simulink model "BEV_PTC"  (R2023a)
settings: Solver=ode23tb  StartTime=0.0  StopTime=20e3  MaxStep=1  RelTol=1e-3
values from neighbouring files (symbols this model uses):
  mass = 20e3    (= 20000)    [run_BEV_simulations.m]    (also in run_FCHEV_simulations.m)
libraries: component_lib x67, slpidlib x6
settings Model: Creator=maxjo  LastModifiedBy=maxjo
settings SolverCC: ZeroCrossControl=DisableAll

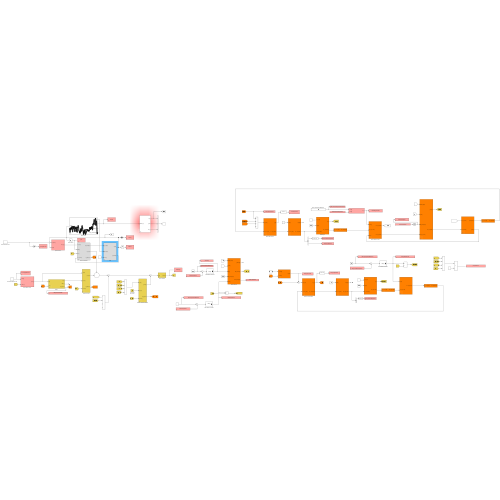
[thumbnail: Simulink's stored preview of the top-level diagram]
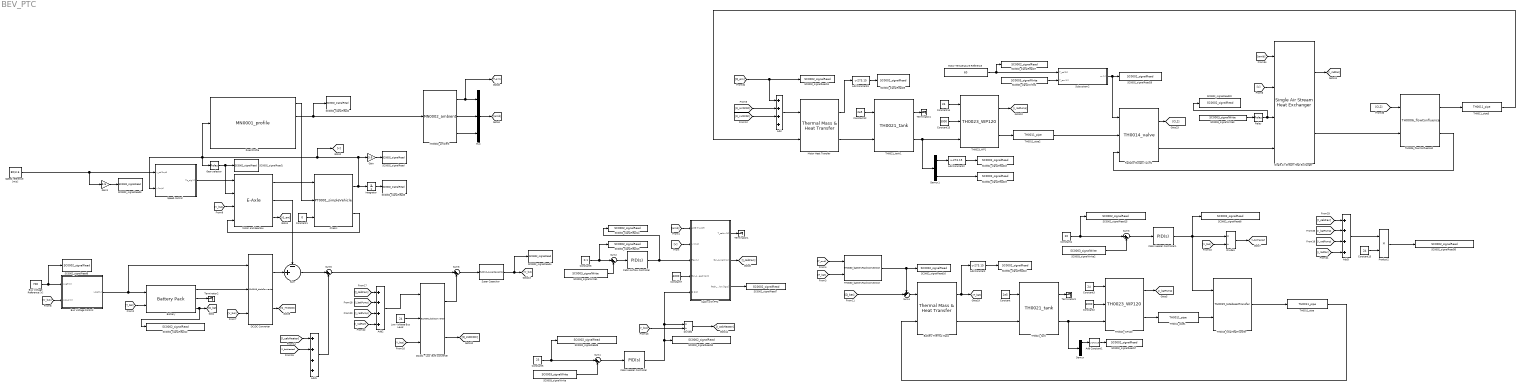
== system BEV_PTC ==
  Add{,1..3} (4 alike) : Sum  Inputs=++++
  Add Constant{,1..3} (4 alike) : Bias  Bias=-273.15  SaturateOnIntegerOverflow=off
  Battery : component_lib/Battery Pack  SOC_0=0.9  Nx=250  Ny=180
  Battery Thermal Mass : component_lib/Thermal Mass & Heat Transfer  n=100  d=10e-3  L=4  m=250 * 180 * 0.048  cp=1040  T_0=273 + 20
  Bus Voltage Control : Subsystem
  Bus Voltage Reference [V] : Constant  Value=700
  Cabin Airflow Controller : slpidlib/PID Controller  Controller=PID  Form=Parallel  TimeDomain=Continuous-time  UseExternalTs=off  SampleTime=-1  IntegratorMethod=Forward Euler  FilterMethod=Forward Euler  ControllerParametersSource=internal  P=1  I=1e-1  UseKiTs=off  D=0  N=100  UseFilter=on  TunerSelectOption=Transfer Function Based (PID Tuner App)  ZeroCross=off  InitialConditionSource=internal  InitialConditionForIntegrator=0.5  InitialConditionForFilter=0  DifferentiatorICPrevScaledInput=0  ExternalReset=none  TrackingMode=off  Kt=1  LimitOutput=on  SatLimitsSource=internal  UpperSaturationLimit=1  LowerSaturationLimit=0  LinearizeAsGain=on  AntiWindupMode=clamping  Kb=1  LimitIntegrator=off  UpperIntegratorSaturationLimit=inf  LowerIntegratorSaturationLimit=-inf  POutMin=[]  POutMax=[]  IOutMin=[]  IOutMax=[]  DOutMin=[]  DOutMax=[]  NOutMin=[]  NOutMax=[]  SumOutMin=[]  SumOutMax=[]  SaturationOutMin=[]  SaturationOutMax=[]  PParamMin=[]  PParamMax=[]  IParamMin=[]  IParamMax=[]  DParamMin=[]  DParamMax=[]  NParamMin=[]  NParamMax=[]  KbParamMin=[]  KbParamMax=[]  KtParamMin=[]  KtParamMax=[]  KbOutMin=[]  KbOutMax=[]  KtOutMin=[]  KtOutMax=[]  IntegratorOutMin=[]  IntegratorOutMax=[]  FilterOutMin=[]  FilterOutMax=[]  SumI1OutMin=[]  SumI1OutMax=[]  SumI2OutMin=[]  SumI2OutMax=[]  SumI3OutMin=[]  SumI3OutMax=[]  SumI4OutMin=[]  SumI4OutMax=[]  SumDOutMin=[]  SumDOutMax=[]  DifferentiatorOutMin=[]  DifferentiatorOutMax=[]  FilterDiffOutCoefMin=[]  FilterDiffOutCoefMax=[]  ReciprocalOutMin=[]  ReciprocalOutMax=[]  SumDenOutMin=[]  SumDenOutMax=[]  SumNumOutMin=[]  SumNumOutMax=[]  DivideOutMin=[]  DivideOutMax=[]  UdiffTsProdOutMin=[]  UdiffTsProdOutMax=[]  NTsProdOutMin=[]  NTsProdOutMax=[]  UintegralTsProdOutMin=[]  UintegralTsProdOutMax=[]  UngainTsProdOutMin=[]  UngainTsProdOutMax=[]  ClampingZeroOutDataTypeStr=Inherit: Inherit via back propagation  ClampingZeroOutMin=[]  ClampingZeroOutMax=[]  FilterDenConstantOutDataTypeStr=Inherit: Inherit via back propagation  FilterDenConstantOutMin=[]  FilterDenConstantOutMax=[]  PCopyOutDataTypeStr=Inherit: Inherit via back propagation  PCopyOutMin=[]  PCopyOutMax=[]  NCopyOutDataTypeStr=Inherit: Inherit via back propagation  NCopyOutMin=[]  NCopyOutMax=[]  IntegratorContinuousStateAttributes=''  IntegratorStateMustResolveToSignalObject=off  IntegratorRTWStateStorageClass=Auto  FilterContinuousStateAttributes=''  FilterStateMustResolveToSignalObject=off  FilterRTWStateStorageClass=Auto  ParallelPVariant=InternalParameters  IdealPVariant=Disabled  IVariant=InternalParameters  DVariant=InternalParameters  IntegratorVariant=Continuous  SatVariant=Enabled  AWVariant=ContClampingParallel  PCopyVariant=Disabled  TRVariant=Disabled  FdbkBlocksVariant=Forward  IdealPFdbkVariant=Disabled  SatFdbkVariant=Disabled  DerivativeFilterVariant=ContFilter  NVariant=InternalParameters  NCopyVariant=Disabled  FilterICVariant=InternalICsFilter  IntegratorICVariant=InternalICs  ExternalResetVariant=Disabled  TRSumVariant=Passthrough  SumFdbkVariant=Disabled  SumVariant=Sum_PID  TsampFilterVariant=InternalTs  TsampNgainVariant=Passthrough  TsampIntegralVariant=Disabled_SignalSpec  ExternalSaturationOutDataTypeStr=Inherit: Same as second input
  Cabin Heater Controller : slpidlib/PID Controller  Controller=PID  Form=Parallel  TimeDomain=Continuous-time  UseExternalTs=off  SampleTime=-1  IntegratorMethod=Forward Euler  FilterMethod=Forward Euler  ControllerParametersSource=internal  P=1e2  I=1e1  UseKiTs=off  D=0  N=100  UseFilter=on  TunerSelectOption=Transfer Function Based (PID Tuner App)  ZeroCross=off  InitialConditionSource=internal  InitialConditionForIntegrator=0  InitialConditionForFilter=0  DifferentiatorICPrevScaledInput=0  ExternalReset=none  TrackingMode=off  Kt=1  LimitOutput=on  SatLimitsSource=internal  UpperSaturationLimit=inf  LowerSaturationLimit=0  LinearizeAsGain=on  AntiWindupMode=clamping  Kb=1  LimitIntegrator=off  UpperIntegratorSaturationLimit=inf  LowerIntegratorSaturationLimit=-inf  POutMin=[]  POutMax=[]  IOutMin=[]  IOutMax=[]  DOutMin=[]  DOutMax=[]  NOutMin=[]  NOutMax=[]  SumOutMin=[]  SumOutMax=[]  SaturationOutMin=[]  SaturationOutMax=[]  PParamMin=[]  PParamMax=[]  IParamMin=[]  IParamMax=[]  DParamMin=[]  DParamMax=[]  NParamMin=[]  NParamMax=[]  KbParamMin=[]  KbParamMax=[]  KtParamMin=[]  KtParamMax=[]  KbOutMin=[]  KbOutMax=[]  KtOutMin=[]  KtOutMax=[]  IntegratorOutMin=[]  IntegratorOutMax=[]  FilterOutMin=[]  FilterOutMax=[]  SumI1OutMin=[]  SumI1OutMax=[]  SumI2OutMin=[]  SumI2OutMax=[]  SumI3OutMin=[]  SumI3OutMax=[]  SumI4OutMin=[]  SumI4OutMax=[]  SumDOutMin=[]  SumDOutMax=[]  DifferentiatorOutMin=[]  DifferentiatorOutMax=[]  FilterDiffOutCoefMin=[]  FilterDiffOutCoefMax=[]  ReciprocalOutMin=[]  ReciprocalOutMax=[]  SumDenOutMin=[]  SumDenOutMax=[]  SumNumOutMin=[]  SumNumOutMax=[]  DivideOutMin=[]  DivideOutMax=[]  UdiffTsProdOutMin=[]  UdiffTsProdOutMax=[]  NTsProdOutMin=[]  NTsProdOutMax=[]  UintegralTsProdOutMin=[]  UintegralTsProdOutMax=[]  UngainTsProdOutMin=[]  UngainTsProdOutMax=[]  ClampingZeroOutDataTypeStr=Inherit: Inherit via back propagation  ClampingZeroOutMin=[]  ClampingZeroOutMax=[]  FilterDenConstantOutDataTypeStr=Inherit: Inherit via back propagation  FilterDenConstantOutMin=[]  FilterDenConstantOutMax=[]  PCopyOutDataTypeStr=Inherit: Inherit via back propagation  PCopyOutMin=[]  PCopyOutMax=[]  NCopyOutDataTypeStr=Inherit: Inherit via back propagation  NCopyOutMin=[]  NCopyOutMax=[]  IntegratorContinuousStateAttributes=''  IntegratorStateMustResolveToSignalObject=off  IntegratorRTWStateStorageClass=Auto  FilterContinuousStateAttributes=''  FilterStateMustResolveToSignalObject=off  FilterRTWStateStorageClass=Auto  ParallelPVariant=InternalParameters  IdealPVariant=Disabled  IVariant=InternalParameters  DVariant=InternalParameters  IntegratorVariant=Continuous  SatVariant=Enabled  AWVariant=ContClampingParallel  PCopyVariant=Disabled  TRVariant=Disabled  FdbkBlocksVariant=Forward  IdealPFdbkVariant=Disabled  SatFdbkVariant=Disabled  DerivativeFilterVariant=ContFilter  NVariant=InternalParameters  NCopyVariant=Disabled  FilterICVariant=InternalICsFilter  IntegratorICVariant=InternalICs  ExternalResetVariant=Disabled  TRSumVariant=Passthrough  SumFdbkVariant=Disabled  SumVariant=Sum_PID  TsampFilterVariant=InternalTs  TsampNgainVariant=Passthrough  TsampIntegralVariant=Disabled_SignalSpec  ExternalSaturationOutDataTypeStr=Inherit: Same as second input
  Cabin Heater Controller1 : slpidlib/PID Controller  Controller=PID  Form=Parallel  TimeDomain=Continuous-time  UseExternalTs=off  SampleTime=-1  IntegratorMethod=Forward Euler  FilterMethod=Forward Euler  ControllerParametersSource=internal  P=1e2  I=1e1  UseKiTs=off  D=0  N=100  UseFilter=on  TunerSelectOption=Transfer Function Based (PID Tuner App)  ZeroCross=off  InitialConditionSource=internal  InitialConditionForIntegrator=0  InitialConditionForFilter=0  DifferentiatorICPrevScaledInput=0  ExternalReset=none  TrackingMode=off  Kt=1  LimitOutput=on  SatLimitsSource=internal  UpperSaturationLimit=inf  LowerSaturationLimit=0  LinearizeAsGain=on  AntiWindupMode=clamping  Kb=1  LimitIntegrator=off  UpperIntegratorSaturationLimit=inf  LowerIntegratorSaturationLimit=-inf  POutMin=[]  POutMax=[]  IOutMin=[]  IOutMax=[]  DOutMin=[]  DOutMax=[]  NOutMin=[]  NOutMax=[]  SumOutMin=[]  SumOutMax=[]  SaturationOutMin=[]  SaturationOutMax=[]  PParamMin=[]  PParamMax=[]  IParamMin=[]  IParamMax=[]  DParamMin=[]  DParamMax=[]  NParamMin=[]  NParamMax=[]  KbParamMin=[]  KbParamMax=[]  KtParamMin=[]  KtParamMax=[]  KbOutMin=[]  KbOutMax=[]  KtOutMin=[]  KtOutMax=[]  IntegratorOutMin=[]  IntegratorOutMax=[]  FilterOutMin=[]  FilterOutMax=[]  SumI1OutMin=[]  SumI1OutMax=[]  SumI2OutMin=[]  SumI2OutMax=[]  SumI3OutMin=[]  SumI3OutMax=[]  SumI4OutMin=[]  SumI4OutMax=[]  SumDOutMin=[]  SumDOutMax=[]  DifferentiatorOutMin=[]  DifferentiatorOutMax=[]  FilterDiffOutCoefMin=[]  FilterDiffOutCoefMax=[]  ReciprocalOutMin=[]  ReciprocalOutMax=[]  SumDenOutMin=[]  SumDenOutMax=[]  SumNumOutMin=[]  SumNumOutMax=[]  DivideOutMin=[]  DivideOutMax=[]  UdiffTsProdOutMin=[]  UdiffTsProdOutMax=[]  NTsProdOutMin=[]  NTsProdOutMax=[]  UintegralTsProdOutMin=[]  UintegralTsProdOutMax=[]  UngainTsProdOutMin=[]  UngainTsProdOutMax=[]  ClampingZeroOutDataTypeStr=Inherit: Inherit via back propagation  ClampingZeroOutMin=[]  ClampingZeroOutMax=[]  FilterDenConstantOutDataTypeStr=Inherit: Inherit via back propagation  FilterDenConstantOutMin=[]  FilterDenConstantOutMax=[]  PCopyOutDataTypeStr=Inherit: Inherit via back propagation  PCopyOutMin=[]  PCopyOutMax=[]  NCopyOutDataTypeStr=Inherit: Inherit via back propagation  NCopyOutMin=[]  NCopyOutMax=[]  IntegratorContinuousStateAttributes=''  IntegratorStateMustResolveToSignalObject=off  IntegratorRTWStateStorageClass=Auto  FilterContinuousStateAttributes=''  FilterStateMustResolveToSignalObject=off  FilterRTWStateStorageClass=Auto  ParallelPVariant=InternalParameters  IdealPVariant=Disabled  IVariant=InternalParameters  DVariant=InternalParameters  IntegratorVariant=Continuous  SatVariant=Enabled  AWVariant=ContClampingParallel  PCopyVariant=Disabled  TRVariant=Disabled  FdbkBlocksVariant=Forward  IdealPFdbkVariant=Disabled  SatFdbkVariant=Disabled  DerivativeFilterVariant=ContFilter  NVariant=InternalParameters  NCopyVariant=Disabled  FilterICVariant=InternalICsFilter  IntegratorICVariant=InternalICs  ExternalResetVariant=Disabled  TRSumVariant=Passthrough  SumFdbkVariant=Disabled  SumVariant=Sum_PID  TsampFilterVariant=InternalTs  TsampNgainVariant=Passthrough  TsampIntegralVariant=Disabled_SignalSpec  ExternalSaturationOutDataTypeStr=Inherit: Same as second input
  Cabin with PTC : Subsystem
  Chassi : component_lib/Powertrain/PT0001_simpleVehicle  m=mass  r_w=0.5  A_f=10  C_d=0.5  rho_air=1.225  c_r0=0.0060  c_r1=2.3e-7  gain=600  v0=75/3.6  x0=0
  Constant : Constant  Value=2e5
  Constant1 : Constant  Value=0
  Constant12 : Constant  Value=2e5
  Constant13 : Constant  Value=3000
  Constant14 : Constant  Value=24
  Constant15 : Constant  Value=24
  Constant2 : Constant  Value=3000
  Constant3 : Constant  Value=24
  Constant4 : Constant  Value=20
  Constant5 : Constant  Value=23
  Constant6 : Constant  Value=0.1
  Constant7 : Constant  Value=4000
  DC/DC - Low level converter : component_lib/Electrochemistry/EL0008_dcdcConverter  eta_up=0.98  eta_down=0.98
  DC/DC Converter : component_lib/Electrochemistry/EL0008_dcdcConverter  eta_up=0.99  eta_down=0.99
  Demux : Demux  Outputs=3
  Demux1 : Demux  Outputs=3
  Divide1 : Product  Inputs=*/
  Divide2 : Product  Inputs=*/
  Gain : Gain  Gain=3.6
  Gain1 : Gain  Gain=3.6
  Gear selector : Relay  OnSwitchValue=22  OffSwitchValue=21.5  OnOutputValue=4  OffOutputValue=3
  Integrator : Integrator
  Low Voltage Bus Level : Constant  Value=24
  MN0002_ambient : component_lib/Mission/MN0002_ambient  p_0=1.01e5  T_0=T_amb  RH_0=0.2
  Motor Heat Transfer : component_lib/Thermal Mass & Heat Transfer  n=100*4  d=10e-3  L=0.6  m=400  cp=420  T_0=273 + 70
  Motor Temperature Reference : Constant  Value=60
  Motor and Gearbox : component_lib/E-Axle  n=4  V_nom=700
  Mux : Mux  Inputs=3
  Product2 : Product
  Radiator Bypass Valve1 : component_lib/Thermal Systems/TH0014_valve  d=10e-2  dr=5e-2  C_d=0.9
  Relay : Relay  OnSwitchValue=85  OffSwitchValue=75  OnOutputValue=3000  ZeroCross=off
  Road Profile : component_lib/Mission/MN0001_profile  profile=Sodertalje_Norrkoping.mat  x0=0  N_lookahead=100
  SC0002_signalRead : component_lib/Data & Control/SC0002_signalRead  SigName=velocity
  SC0002_signalRead1 : component_lib/Data & Control/SC0002_signalRead  SigName=gear
  SC0002_signalRead10 : component_lib/Data & Control/SC0002_signalRead  SigName=cabinHeaterPower
  SC0002_signalRead11 : component_lib/Data & Control/SC0002_signalRead  SigName=motorGeneratedHeat
  SC0002_signalRead12 : component_lib/Data & Control/SC0002_signalRead  SigName=batteryGeneratedHeat
  SC0002_signalRead13 : component_lib/Data & Control/SC0002_signalRead  SigName=cabinFreshAirFlowReference
  SC0002_signalRead14 : component_lib/Data & Control/SC0002_signalRead  SigName=cabinFlap
  SC0002_signalRead15 : component_lib/Data & Control/SC0002_signalRead  SigName=batteryTemperatureReference
  SC0002_signalRead16 : component_lib/Data & Control/SC0002_signalRead  SigName=batteryConvection
  SC0002_signalRead17 : component_lib/Data & Control/SC0002_signalRead  SigName=batteryCoolantTemperature
  SC0002_signalRead18 : component_lib/Data & Control/SC0002_signalRead  SigName=radiatorCoolantTemperature
  SC0002_signalRead19 : component_lib/Data & Control/SC0002_signalRead  SigName=radiatorCoolantFlow
  SC0002_signalRead2 : component_lib/Data & Control/SC0002_signalRead  SigName=altitude
  SC0002_signalRead20 : component_lib/Data & Control/SC0002_signalRead  SigName=radiatorFanSpeed
  SC0002_signalRead22 : component_lib/Data & Control/SC0002_signalRead  SigName=batteryTemperature
  SC0002_signalRead25 : component_lib/Data & Control/SC0002_signalRead  SigName=motorTemperature
  SC0002_signalRead26 : component_lib/Data & Control/SC0002_signalRead  SigName=radiatorBypassValve
  SC0002_signalRead27 : component_lib/Data & Control/SC0002_signalRead  SigName=radiatorCoolantTemperatureReference
  SC0002_signalRead3 : component_lib/Data & Control/SC0002_signalRead  SigName=velocityReference
  SC0002_signalRead30 : component_lib/Data & Control/SC0002_signalRead  SigName=pumpfanPower
  SC0002_signalRead4 : component_lib/Data & Control/SC0002_signalRead  SigName=busVoltage
  SC0002_signalRead5 : component_lib/Data & Control/SC0002_signalRead  SigName=distance
  SC0002_signalRead6 : component_lib/Data & Control/SC0002_signalRead  SigName=busVoltageReference
  SC0002_signalRead7 : component_lib/Data & Control/SC0002_signalRead  SigName=cabinFreshAirFlow
  SC0002_signalRead8 : component_lib/Data & Control/SC0002_signalRead  SigName=batteryHeaterPower
  SC0002_signalRead9 : component_lib/Data & Control/SC0002_signalRead  SigName=cabinTemperatureReference
  SC0003_signalWrite : component_lib/Data & Control/SC0003_signalWrite  SigName=cabinTemperature
  SC0003_signalWrite1 : component_lib/Data & Control/SC0003_signalWrite  SigName=cabinFreshAirFlow
  SC0003_signalWrite2 : component_lib/Data & Control/SC0003_signalWrite  SigName=batteryCoolantTemperature
  SC0003_signalWrite3 : component_lib/Data & Control/SC0003_signalWrite  SigName=motorTemperature
  SC0003_signalWrite4 : component_lib/Data & Control/SC0003_signalWrite  SigName=radiatorCoolantTemperature
  Single Air Stream Heat Exchanger : component_lib/Single Air Stream Heat Exchanger  HtH=1.1  StS=0.95
  Speed control : Subsystem
  Speed reference [m/s] : Constant  Value=80/3.6
  Subsystem2 : Subsystem
  Sum : Sum  Inputs=-+|
  Sum{1..3,5..6} (5 alike) : Sum  Inputs=|+-
  Sum4 : Sum  Inputs=++|
  Super Capacitor : component_lib/Electrochemistry/EL0010_superCapacitor  C=100  V_bus0=700
  TH0006_flowConfluence2 : component_lib/Thermal Systems/TH0006_flowConfluence  gain=0.01
  TH0011_pipe : component_lib/Thermal Systems/TH0011_pipe  d=19e-3  L=5  e=0.006e-3  T_0=273 + 20
  TH0011_pipe1 : component_lib/Thermal Systems/TH0011_pipe  d=19e-3  L=2  e=0.006e-3  T_0=273 + 20
  TH0011_pipe2 : component_lib/Thermal Systems/TH0011_pipe  d=19e-3  L=2  e=0.006e-3  T_0=273 + 20
  TH0011_pipe3 : component_lib/Thermal Systems/TH0011_pipe  d=19e-3  L=5  e=0.006e-3  T_0=273 + 20
  TH0015_totalHeatTransfer : component_lib/Thermal Systems/TH0015_totalHeatTransfer  T_max=273+100  T_min=273
  TH0021_tank : component_lib/Thermal Systems/TH0021_tank  V=5e-3  T0=273.15 + 25
  TH0021_tank1 : component_lib/Thermal Systems/TH0021_tank  V=5e-3  T0=273.15 + 25
  TH0023_WP1 : component_lib/Thermal Systems/TH0023_WP120  SystemSampleTime=-1  VariantActivationTime=update diagram  Latency=0  AutoFrameSizeCalculation=off
  TH0023_WP120 : component_lib/Thermal Systems/TH0023_WP120  SystemSampleTime=-1  VariantActivationTime=update diagram  Latency=0  AutoFrameSizeCalculation=off
  TH0030_batteryPackConvection : component_lib/Thermal Systems/TH0030_batteryPackConvection  A=2*10  h=8
  Terminator{1..4} (4 alike) : Terminator
  wires:
  Speed reference [m/s]/1 -> Speed control/1(v_ref [m/s]), Gain1/1
  Motor and Gearbox/2 -> Sum/1
  Bus Voltage Reference [V]/1 -> Bus Voltage Control/1(V_ref [V]), SC0002_signalRead6/1
  Chassi/1 -> Integrator/1, Gain/1, [v], Speed control/2(v [m/s]), Road Profile/1, Gear selector/1
  Battery/2 -> Terminator2/1
  Motor and Gearbox/1 -> Chassi/1
  DC/DC Converter/1 -> Sum/2
  Road Profile/1 -> Chassi/2
  Road Profile/2 -> MN0002_ambient/1, SC0002_signalRead2/1
  Constant1/1 -> Chassi/3
  [T_bat] -> Battery/2
  Gain/1 -> SC0002_signalRead/1
  Gear selector/1 -> Motor and Gearbox/2, SC0002_signalRead1/1
  Gain1/1 -> SC0002_signalRead3/1
  Chassi/2 -> Motor and Gearbox/4
  Bus Voltage Control/1(I_bat [-]) -> DC/DC Converter/1, Battery/1
  Integrator/1 -> SC0002_signalRead5/1
  Speed control/1(Tq_sig [-]) -> Motor and Gearbox/1
  Super Capacitor/1 -> [V_bus], SC0002_signalRead4/1
  Battery/1 -> DC/DC Converter/2
  Battery/3 -> SC0002_signalRead12/1, [Q_bat]
  Motor and Gearbox/3 -> [Q_em]
  Cabin Airflow Controller/1 -> Cabin with PTC/3(flap [-]), SC0002_signalRead14/1
  Constant7/1 -> Cabin with PTC/4(fan_speed [rpm])
  [v] -> Cabin with PTC/2(v [m/s])
  MN0002_ambient/3 -> Mux/3
  MN0002_ambient/1 -> [T_amb], Mux/1
  MN0002_ambient/2 -> Mux/2
  Mux/1 -> [amb]
  [amb] -> Cabin with PTC/1(AMB (T,p,RH))
  Cabin with PTC/3(fresh_flow [kg/s]) -> SC0002_signalRead7/1
  Constant5/1 -> Sum1/1, SC0002_signalRead9/1
  SC0003_signalWrite/1 -> Sum1/2
  Sum1/1 -> Cabin Heater Controller/1
  SC0003_signalWrite1/1 -> Sum2/2
  Sum2/1 -> Cabin Airflow Controller/1
  Constant6/1 -> Sum2/1, SC0002_signalRead13/1
  Cabin with PTC/1(T_cabin [K]) -> Terminator1/1
  Cabin with PTC/2(fan_current [A]) -> [I_cabFan]
  Cabin Heater Controller/1 -> Divide2/1, Cabin with PTC/5(Q [J/s]), SC0002_signalRead10/1
  Battery Thermal Mass/1 -> [T_bat], Add Constant/1
  TH0015_totalHeatTransfer/1 -> TH0011_pipe/1
  TH0011_pipe1/1 -> TH0015_totalHeatTransfer/2
  Constant/1 -> TH0021_tank/1
  TH0021_tank/2 -> Demux/1, TH0023_WP120/3
  TH0023_WP120/2 -> TH0011_pipe1/1
  Battery Thermal Mass/2 -> TH0021_tank/2
  Constant2/1 -> TH0023_WP120/2
  Constant3/1 -> TH0023_WP120/1
  TH0023_WP120/1 -> [I_batPump]
  SC0003_signalWrite2/1 -> Sum3/2
  Divide1/1 -> [I_batHeater]
  Cabin Heater Controller1/1 -> SC0002_signalRead8/1, TH0015_totalHeatTransfer/1, Divide1/1
  Sum3/1 -> Cabin Heater Controller1/1
  Constant4/1 -> Sum3/1, SC0002_signalRead15/1
  TH0021_tank/1 -> Terminator3/1
  Add Constant/1 -> SC0002_signalRead22/1
  [T_bat] -> TH0030_batteryPackConvection/2
  [T_amb] -> TH0030_batteryPackConvection/1
  [Q_bat] -> Sum4/2
  Sum4/1 -> Battery Thermal Mass/1
  TH0030_batteryPackConvection/1 -> SC0002_signalRead16/1, Sum4/1
  TH0011_pipe/1 -> Battery Thermal Mass/2
  Demux/1 -> Add Constant1/1
  Add Constant1/1 -> SC0002_signalRead17/1
  Radiator Bypass Valve1/1 -> [CL2]
  [CL2] -> TH0006_flowConfluence2/1
  [amb] -> Single Air Stream Heat Exchanger/1
  Motor Temperature Reference/1 -> SC0002_signalRead27/1, Subsystem2/1(T_ref [K])
  TH0011_pipe3/1 -> Motor Heat Transfer/2
  Subsystem2/1(cv [-]) -> Radiator Bypass Valve1/1, SC0002_signalRead26/1
  SC0003_signalWrite4/1 -> Subsystem2/2(T_em [K])
  TH0011_pipe2/1 -> Radiator Bypass Valve1/2
  Motor Heat Transfer/1 -> Add Constant3/1
  DC/DC Converter/2 -> [Q_HVDCDC]
  TH0023_WP1/2 -> TH0011_pipe2/1
  Add Constant2/1 -> SC0002_signalRead18/1
  Constant12/1 -> TH0021_tank1/1
  Constant14/1 -> TH0023_WP1/1
  TH0021_tank1/1 -> Terminator4/1
  TH0021_tank1/2 -> Demux1/1, TH0023_WP1/3
  TH0023_WP1/1 -> [I_radPump]
  Constant13/1 -> TH0023_WP1/2
  Demux1/1 -> Add Constant2/1
  Motor Heat Transfer/2 -> TH0021_tank1/2
  Add Constant3/1 -> SC0002_signalRead25/1
  TH0006_flowConfluence2/2 -> Radiator Bypass Valve1/3
  Radiator Bypass Valve1/2 -> Single Air Stream Heat Exchanger/4
  Single Air Stream Heat Exchanger/2 -> TH0006_flowConfluence2/2
  [v] -> Single Air Stream Heat Exchanger/2
  Single Air Stream Heat Exchanger/1 -> [I_radFan]
  Demux1/3 -> SC0002_signalRead19/1
  Relay/1 -> SC0002_signalRead20/1, Single Air Stream Heat Exchanger/3
  SC0003_signalWrite3/1 -> Relay/1
  [Q_em] -> SC0002_signalRead11/1, Add/1
  [V_bus] -> DC/DC - Low level converter/3
  Low Voltage Bus Level/1 -> DC/DC - Low level converter/2
  DC/DC - Low level converter/1 -> Sum6/2
  DC/DC - Low level converter/2 -> [Q_LVDCDC]
  Sum6/1 -> Super Capacitor/1
  [V_bus] -> DC/DC Converter/3
  [V_bus] -> Bus Voltage Control/2(V_bus [V])
  [V_bus] -> Motor and Gearbox/3
  Add/1 -> Motor Heat Transfer/1
  [Q_HVDCDC] -> Add/2
  [Q_LVDCDC] -> Add/3
  [V_bus] -> Divide1/2
  [V_bus] -> Divide2/2
  Divide2/1 -> [I_cabHeater]
  Sum/1 -> Sum5/1
  Sum5/1 -> Sum6/1
  Add1/1 -> Sum5/2
  [I_cabHeater] -> Add1/1
  [I_batHeater] -> Add1/2
  Add2/1 -> DC/DC - Low level converter/1
  [I_cabFan] -> Add2/1
  [I_batPump] -> Add2/2
  Add3/1 -> Product2/1
  [I_radPump] -> Add3/3
  [I_cabFan] -> Add3/1
  Product2/1 -> SC0002_signalRead30/1
  Constant15/1 -> Product2/2
  [I_batPump] -> Add3/2
  [I_radPump] -> Add2/3
  TH0006_flowConfluence2/1 -> TH0011_pipe3/1
  [I_radFan] -> Add3/4
  [I_radFan] -> Add2/4

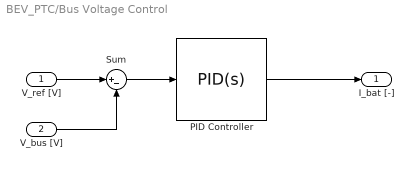
== system BEV_PTC/Bus Voltage Control ==
  V_ref [V] : Inport
  V_bus [V] : Inport  Port=2
  PID Controller : slpidlib/PID Controller  Controller=PID  Form=Parallel  TimeDomain=Continuous-time  UseExternalTs=off  SampleTime=-1  IntegratorMethod=Forward Euler  FilterMethod=Forward Euler  ControllerParametersSource=internal  P=1e2  I=1  UseKiTs=off  D=0  N=100  UseFilter=on  TunerSelectOption=Transfer Function Based (PID Tuner App)  ZeroCross=off  InitialConditionSource=internal  InitialConditionForIntegrator=0  InitialConditionForFilter=0  DifferentiatorICPrevScaledInput=0  ExternalReset=none  TrackingMode=off  Kt=1  LimitOutput=on  SatLimitsSource=internal  UpperSaturationLimit=725*2  LowerSaturationLimit=-725  LinearizeAsGain=on  AntiWindupMode=clamping  Kb=1  LimitIntegrator=off  UpperIntegratorSaturationLimit=inf  LowerIntegratorSaturationLimit=-inf  POutMin=[]  POutMax=[]  IOutMin=[]  IOutMax=[]  DOutMin=[]  DOutMax=[]  NOutMin=[]  NOutMax=[]  SumOutMin=[]  SumOutMax=[]  SaturationOutMin=[]  SaturationOutMax=[]  PParamMin=[]  PParamMax=[]  IParamMin=[]  IParamMax=[]  DParamMin=[]  DParamMax=[]  NParamMin=[]  NParamMax=[]  KbParamMin=[]  KbParamMax=[]  KtParamMin=[]  KtParamMax=[]  KbOutMin=[]  KbOutMax=[]  KtOutMin=[]  KtOutMax=[]  IntegratorOutMin=[]  IntegratorOutMax=[]  FilterOutMin=[]  FilterOutMax=[]  SumI1OutMin=[]  SumI1OutMax=[]  SumI2OutMin=[]  SumI2OutMax=[]  SumI3OutMin=[]  SumI3OutMax=[]  SumI4OutMin=[]  SumI4OutMax=[]  SumDOutMin=[]  SumDOutMax=[]  DifferentiatorOutMin=[]  DifferentiatorOutMax=[]  FilterDiffOutCoefMin=[]  FilterDiffOutCoefMax=[]  ReciprocalOutMin=[]  ReciprocalOutMax=[]  SumDenOutMin=[]  SumDenOutMax=[]  SumNumOutMin=[]  SumNumOutMax=[]  DivideOutMin=[]  DivideOutMax=[]  UdiffTsProdOutMin=[]  UdiffTsProdOutMax=[]  NTsProdOutMin=[]  NTsProdOutMax=[]  UintegralTsProdOutMin=[]  UintegralTsProdOutMax=[]  UngainTsProdOutMin=[]  UngainTsProdOutMax=[]  ClampingZeroOutDataTypeStr=Inherit: Inherit via back propagation  ClampingZeroOutMin=[]  ClampingZeroOutMax=[]  FilterDenConstantOutDataTypeStr=Inherit: Inherit via back propagation  FilterDenConstantOutMin=[]  FilterDenConstantOutMax=[]  PCopyOutDataTypeStr=Inherit: Inherit via back propagation  PCopyOutMin=[]  PCopyOutMax=[]  NCopyOutDataTypeStr=Inherit: Inherit via back propagation  NCopyOutMin=[]  NCopyOutMax=[]  IntegratorContinuousStateAttributes=''  IntegratorStateMustResolveToSignalObject=off  IntegratorRTWStateStorageClass=Auto  FilterContinuousStateAttributes=''  FilterStateMustResolveToSignalObject=off  FilterRTWStateStorageClass=Auto  ParallelPVariant=InternalParameters  IdealPVariant=Disabled  IVariant=InternalParameters  DVariant=InternalParameters  IntegratorVariant=Continuous  SatVariant=Enabled  AWVariant=ContClampingParallel  PCopyVariant=Disabled  TRVariant=Disabled  FdbkBlocksVariant=Forward  IdealPFdbkVariant=Disabled  SatFdbkVariant=Disabled  DerivativeFilterVariant=ContFilter  NVariant=InternalParameters  NCopyVariant=Disabled  FilterICVariant=InternalICsFilter  IntegratorICVariant=InternalICs  ExternalResetVariant=Disabled  TRSumVariant=Passthrough  SumFdbkVariant=Disabled  SumVariant=Sum_PID  TsampFilterVariant=InternalTs  TsampNgainVariant=Passthrough  TsampIntegralVariant=Disabled_SignalSpec  ExternalSaturationOutDataTypeStr=Inherit: Same as second input
  Sum : Sum  Inputs=|+-
  I_bat [-] : Outport
  wires:
  PID Controller/1 -> I_bat [-]/1
  Sum/1 -> PID Controller/1
  V_ref [V]/1 -> Sum/1
  V_bus [V]/1 -> Sum/2

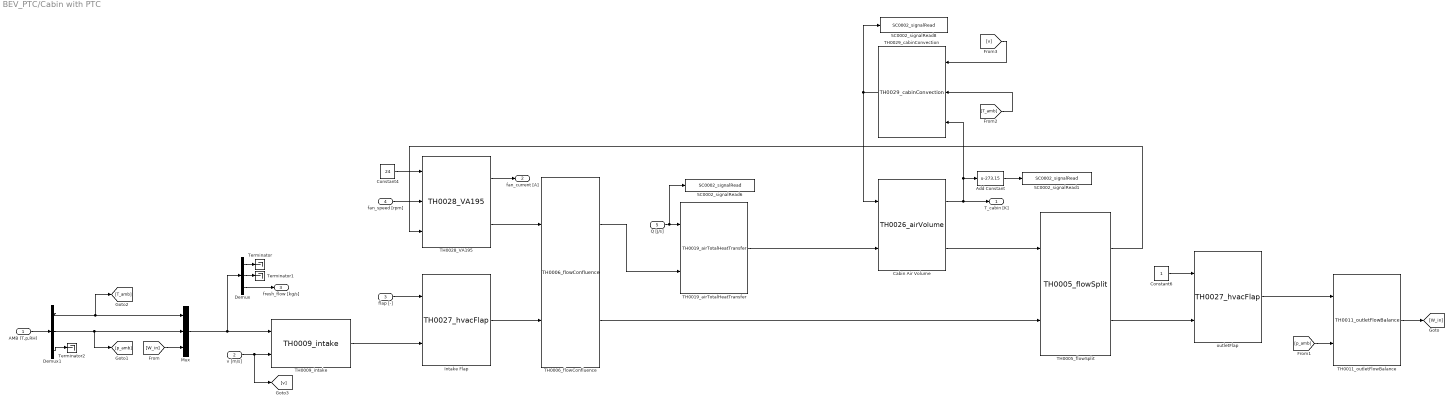
== system BEV_PTC/Cabin with PTC ==
  AMB (T,p,RH) : Inport
  v [m/s] : Inport  Port=2
  flap [-] : Inport  Port=3
  fan_speed [rpm] : Inport  Port=4
  Q [J/s] : Inport  Port=5
  Add Constant : Bias  Bias=-273.15  SaturateOnIntegerOverflow=off
  Cabin Air Volume : component_lib/Thermal Systems/TH0026_airVolume  V=4  T0=273.15 + 20
  Constant4 : Constant  Value=24
  Constant6 : Constant
  Demux : Demux  Outputs=3
  Demux1 : Demux  Outputs=3
  Intake Flap : component_lib/Thermal Systems/TH0027_hvacFlap  A=0.04  zeta=0.3
  Mux : Mux  Inputs=3
  SC0002_signalRead1 : component_lib/Data & Control/SC0002_signalRead  SigName=cabinTemperature
  SC0002_signalRead6 : component_lib/Data & Control/SC0002_signalRead  SigName=cabinHeating
  SC0002_signalRead8 : component_lib/Data & Control/SC0002_signalRead  SigName=cabinConvection
  TH0005_flowSplit : component_lib/Thermal Systems/TH0005_flowSplit  SystemSampleTime=-1  VariantActivationTime=update diagram  Latency=0  AutoFrameSizeCalculation=off
  TH0006_flowConfluence : component_lib/Thermal Systems/TH0006_flowConfluence  gain=0.01
  TH0009_intake : component_lib/Thermal Systems/TH0009_intake  zeta=0.1
  TH0011_outletFlowBalance : component_lib/Thermal Systems/TH0011_outletFlowBalance  gain=0.05
  TH0019_airTotalHeatTransfer : component_lib/Thermal Systems/TH0019_airTotalHeatTransfer  T_min=273-40  T_max=273+140
  TH0028_VA195 : component_lib/Thermal Systems/TH0028_VA195  n=1
      settings: LibrarySourceBlock=component_lib/Thermal Systems/TH0023_WP120
  TH0029_cabinConvection : component_lib/Thermal Systems/TH0029_cabinConvection  A=2
  Terminator : Terminator
  Terminator1 : Terminator
  Terminator2 : Terminator
  outletFlap : component_lib/Thermal Systems/TH0027_hvacFlap  A=0.04  zeta=0.3
  T_cabin [K] : Outport
  fan_current [A] : Outport  Port=2
  fresh_flow [kg/s] : Outport  Port=3
  wires:
  TH0006_flowConfluence/1 -> TH0019_airTotalHeatTransfer/2
  Add Constant/1 -> SC0002_signalRead1/1
  Demux1/3 -> Terminator2/1
  Demux/2 -> Terminator1/1
  Demux/1 -> Terminator/1
  TH0028_VA195/2 -> TH0006_flowConfluence/1
  TH0009_intake/1 -> Intake Flap/2
  Cabin Air Volume/2 -> TH0005_flowSplit/1
  AMB (T,p,RH)/1 -> Demux1/1
  flap [-]/1 -> Intake Flap/1
  Constant4/1 -> TH0028_VA195/1
  fan_speed [rpm]/1 -> TH0028_VA195/2
  Intake Flap/1 -> TH0006_flowConfluence/2
  [T_amb] -> TH0029_cabinConvection/2
  TH0028_VA195/1 -> fan_current [A]/1
  v [m/s]/1 -> TH0009_intake/2, [v]
  TH0019_airTotalHeatTransfer/1 -> Cabin Air Volume/2
  [v] -> TH0029_cabinConvection/1
  Cabin Air Volume/1 -> T_cabin [K]/1, Add Constant/1, TH0029_cabinConvection/3
  TH0005_flowSplit/2 -> outletFlap/2
  TH0006_flowConfluence/2 -> TH0005_flowSplit/2
  TH0029_cabinConvection/1 -> SC0002_signalRead8/1, Cabin Air Volume/1
  TH0005_flowSplit/1 -> TH0028_VA195/3
  Mux/1 -> TH0009_intake/1, Demux/1
  Q [J/s]/1 -> TH0019_airTotalHeatTransfer/1, SC0002_signalRead6/1
  Demux1/2 -> [p_amb], Mux/2
  outletFlap/1 -> TH0011_outletFlowBalance/1
  Demux1/1 -> [T_amb], Mux/1
  [W_in] -> Mux/3
  TH0011_outletFlowBalance/1 -> [W_in]
  Constant6/1 -> outletFlap/1
  [p_amb] -> TH0011_outletFlowBalance/2
  Demux/3 -> fresh_flow [kg/s]/1

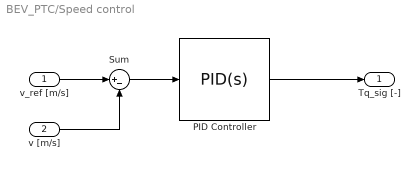
== system BEV_PTC/Speed control ==
  v_ref [m/s] : Inport
  v [m/s] : Inport  Port=2
  PID Controller : slpidlib/PID Controller  Controller=PID  Form=Parallel  TimeDomain=Continuous-time  UseExternalTs=off  SampleTime=-1  IntegratorMethod=Forward Euler  FilterMethod=Forward Euler  ControllerParametersSource=internal  P=10  I=1e-1  UseKiTs=off  D=0  N=100  UseFilter=on  TunerSelectOption=Transfer Function Based (PID Tuner App)  ZeroCross=off  InitialConditionSource=internal  InitialConditionForIntegrator=0  InitialConditionForFilter=0  DifferentiatorICPrevScaledInput=0  ExternalReset=none  TrackingMode=off  Kt=1  LimitOutput=on  SatLimitsSource=internal  UpperSaturationLimit=1  LowerSaturationLimit=-1  LinearizeAsGain=on  AntiWindupMode=clamping  Kb=1  LimitIntegrator=off  UpperIntegratorSaturationLimit=inf  LowerIntegratorSaturationLimit=-inf  POutMin=[]  POutMax=[]  IOutMin=[]  IOutMax=[]  DOutMin=[]  DOutMax=[]  NOutMin=[]  NOutMax=[]  SumOutMin=[]  SumOutMax=[]  SaturationOutMin=[]  SaturationOutMax=[]  PParamMin=[]  PParamMax=[]  IParamMin=[]  IParamMax=[]  DParamMin=[]  DParamMax=[]  NParamMin=[]  NParamMax=[]  KbParamMin=[]  KbParamMax=[]  KtParamMin=[]  KtParamMax=[]  KbOutMin=[]  KbOutMax=[]  KtOutMin=[]  KtOutMax=[]  IntegratorOutMin=[]  IntegratorOutMax=[]  FilterOutMin=[]  FilterOutMax=[]  SumI1OutMin=[]  SumI1OutMax=[]  SumI2OutMin=[]  SumI2OutMax=[]  SumI3OutMin=[]  SumI3OutMax=[]  SumI4OutMin=[]  SumI4OutMax=[]  SumDOutMin=[]  SumDOutMax=[]  DifferentiatorOutMin=[]  DifferentiatorOutMax=[]  FilterDiffOutCoefMin=[]  FilterDiffOutCoefMax=[]  ReciprocalOutMin=[]  ReciprocalOutMax=[]  SumDenOutMin=[]  SumDenOutMax=[]  SumNumOutMin=[]  SumNumOutMax=[]  DivideOutMin=[]  DivideOutMax=[]  UdiffTsProdOutMin=[]  UdiffTsProdOutMax=[]  NTsProdOutMin=[]  NTsProdOutMax=[]  UintegralTsProdOutMin=[]  UintegralTsProdOutMax=[]  UngainTsProdOutMin=[]  UngainTsProdOutMax=[]  ClampingZeroOutDataTypeStr=Inherit: Inherit via back propagation  ClampingZeroOutMin=[]  ClampingZeroOutMax=[]  FilterDenConstantOutDataTypeStr=Inherit: Inherit via back propagation  FilterDenConstantOutMin=[]  FilterDenConstantOutMax=[]  PCopyOutDataTypeStr=Inherit: Inherit via back propagation  PCopyOutMin=[]  PCopyOutMax=[]  NCopyOutDataTypeStr=Inherit: Inherit via back propagation  NCopyOutMin=[]  NCopyOutMax=[]  IntegratorContinuousStateAttributes=''  IntegratorStateMustResolveToSignalObject=off  IntegratorRTWStateStorageClass=Auto  FilterContinuousStateAttributes=''  FilterStateMustResolveToSignalObject=off  FilterRTWStateStorageClass=Auto  ParallelPVariant=InternalParameters  IdealPVariant=Disabled  IVariant=InternalParameters  DVariant=InternalParameters  IntegratorVariant=Continuous  SatVariant=Enabled  AWVariant=ContClampingParallel  PCopyVariant=Disabled  TRVariant=Disabled  FdbkBlocksVariant=Forward  IdealPFdbkVariant=Disabled  SatFdbkVariant=Disabled  DerivativeFilterVariant=ContFilter  NVariant=InternalParameters  NCopyVariant=Disabled  FilterICVariant=InternalICsFilter  IntegratorICVariant=InternalICs  ExternalResetVariant=Disabled  TRSumVariant=Passthrough  SumFdbkVariant=Disabled  SumVariant=Sum_PID  TsampFilterVariant=InternalTs  TsampNgainVariant=Passthrough  TsampIntegralVariant=Disabled_SignalSpec  ExternalSaturationOutDataTypeStr=Inherit: Same as second input
  Sum : Sum  Inputs=|+-
  Tq_sig [-] : Outport
  wires:
  PID Controller/1 -> Tq_sig [-]/1
  Sum/1 -> PID Controller/1
  v_ref [m/s]/1 -> Sum/1
  v [m/s]/1 -> Sum/2

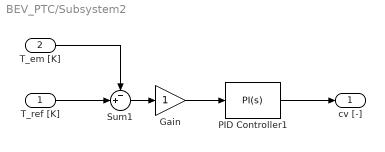
== system BEV_PTC/Subsystem2 ==
  T_ref [K] : Inport
  T_em [K] : Inport  Port=2
  Gain : Gain
  PID Controller1 : slpidlib/PID Controller  Controller=PI  Form=Parallel  TimeDomain=Continuous-time  UseExternalTs=off  SampleTime=-1  IntegratorMethod=Forward Euler  FilterMethod=Forward Euler  ControllerParametersSource=internal  P=1e-1  I=1e-2  UseKiTs=off  D=0  N=100  UseFilter=on  TunerSelectOption=Transfer Function Based (PID Tuner App)  ZeroCross=off  InitialConditionSource=internal  InitialConditionForIntegrator=0.5  InitialConditionForFilter=0.5  DifferentiatorICPrevScaledInput=0  ExternalReset=none  TrackingMode=off  Kt=1  LimitOutput=on  SatLimitsSource=internal  UpperSaturationLimit=0.95  LowerSaturationLimit=0.05  LinearizeAsGain=on  AntiWindupMode=back-calculation  Kb=1  LimitIntegrator=off  UpperIntegratorSaturationLimit=inf  LowerIntegratorSaturationLimit=-inf  POutMin=[]  POutMax=[]  IOutMin=[]  IOutMax=[]  DOutMin=[]  DOutMax=[]  NOutMin=[]  NOutMax=[]  SumOutMin=[]  SumOutMax=[]  SaturationOutMin=[]  SaturationOutMax=[]  PParamMin=[]  PParamMax=[]  IParamMin=[]  IParamMax=[]  DParamMin=[]  DParamMax=[]  NParamMin=[]  NParamMax=[]  KbParamMin=[]  KbParamMax=[]  KtParamMin=[]  KtParamMax=[]  KbOutMin=[]  KbOutMax=[]  KtOutMin=[]  KtOutMax=[]  IntegratorOutMin=[]  IntegratorOutMax=[]  FilterOutMin=[]  FilterOutMax=[]  SumI1OutMin=[]  SumI1OutMax=[]  SumI2OutMin=[]  SumI2OutMax=[]  SumI3OutMin=[]  SumI3OutMax=[]  SumI4OutMin=[]  SumI4OutMax=[]  SumDOutMin=[]  SumDOutMax=[]  DifferentiatorOutMin=[]  DifferentiatorOutMax=[]  FilterDiffOutCoefMin=[]  FilterDiffOutCoefMax=[]  ReciprocalOutMin=[]  ReciprocalOutMax=[]  SumDenOutMin=[]  SumDenOutMax=[]  SumNumOutMin=[]  SumNumOutMax=[]  DivideOutMin=[]  DivideOutMax=[]  UdiffTsProdOutMin=[]  UdiffTsProdOutMax=[]  NTsProdOutMin=[]  NTsProdOutMax=[]  UintegralTsProdOutMin=[]  UintegralTsProdOutMax=[]  UngainTsProdOutMin=[]  UngainTsProdOutMax=[]  ClampingZeroOutDataTypeStr=Inherit: Inherit via back propagation  ClampingZeroOutMin=[]  ClampingZeroOutMax=[]  FilterDenConstantOutDataTypeStr=Inherit: Inherit via back propagation  FilterDenConstantOutMin=[]  FilterDenConstantOutMax=[]  PCopyOutDataTypeStr=Inherit: Inherit via back propagation  PCopyOutMin=[]  PCopyOutMax=[]  NCopyOutDataTypeStr=Inherit: Inherit via back propagation  NCopyOutMin=[]  NCopyOutMax=[]  IntegratorContinuousStateAttributes=''  IntegratorStateMustResolveToSignalObject=off  IntegratorRTWStateStorageClass=Auto  FilterContinuousStateAttributes=''  FilterStateMustResolveToSignalObject=off  FilterRTWStateStorageClass=Auto  ParallelPVariant=InternalParameters  IdealPVariant=Disabled  IVariant=InternalParameters  DVariant=Disabled  IntegratorVariant=Continuous  SatVariant=Enabled  AWVariant=BackCalculation  PCopyVariant=Disabled  TRVariant=Disabled  FdbkBlocksVariant=Forward  IdealPFdbkVariant=Disabled  SatFdbkVariant=Disabled  DerivativeFilterVariant=Disabled  NVariant=Disabled  NCopyVariant=Disabled_SignalSpec  FilterICVariant=Disabled  IntegratorICVariant=InternalICs  ExternalResetVariant=Disabled  TRSumVariant=Passthrough  SumFdbkVariant=Disabled  SumVariant=Sum_PI  TsampFilterVariant=InternalTs  TsampNgainVariant=Passthrough  TsampIntegralVariant=Disabled_SignalSpec  ExternalSaturationOutDataTypeStr=Inherit: Same as second input
  Sum1 : Sum  Inputs=-+|
  cv [-] : Outport
  wires:
  T_em [K]/1 -> Sum1/1
  Gain/1 -> PID Controller1/1
  Sum1/1 -> Gain/1
  PID Controller1/1 -> cv [-]/1
  T_ref [K]/1 -> Sum1/2
